simulink model "VirtualContactAgent"  (Simulink 7.1)
settings: Solver=ode45  StartTime=0.0  StopTime=10.0  RelTol=1e-3
settings Model: Creator=suarezjl  LastModifiedBy=suarezjl

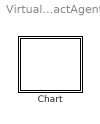
== system VirtualContactAgent ==
  Chart : Stateflow chart

== stateflow chart Chart ==
  state Averaging
    \\Octavia\\ISACControlBasisModule\VirtualContact\VirtualContact.AverageValues()
  state Stop
    \\Octavia\ISACControlBasisModule\VirtualContact\StateMachine.Stop()
  (default) -> Averaging : Start
  Averaging -> Stop : Signal = Stop
